simulink model "StopForInstabilityObserverForce"  (R2016b)
settings: configuration reference "WheelSimConfiguration2016" (kept outside this file)
libraries: simulink x1
settings Model: Creator=At  LastModifiedBy=ateay
settings ConfigSetRef: SourceLocation=Base Workspace

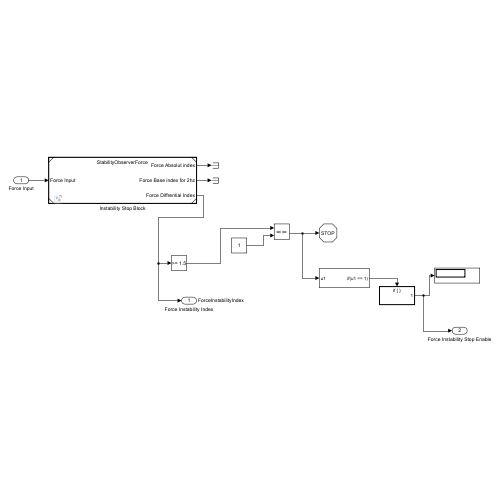
[thumbnail: Simulink's stored preview of the top-level diagram]
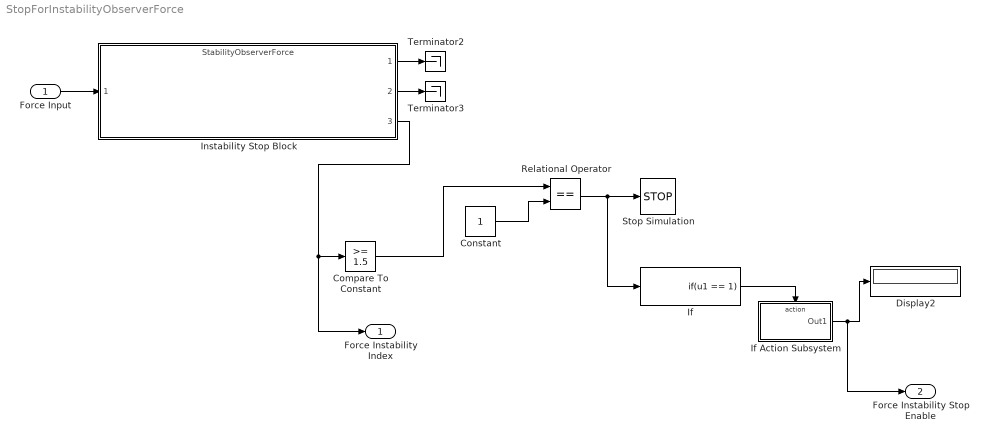
== system StopForInstabilityObserverForce ==
  Force Input : Inport
  Compare To Constant : simulink/Logic and Bit Operations/Compare To Constant  relop=>=  const=1.5  OutDataTypeStr=boolean
  Constant : Constant
  Display2 : Display
  If : If  IfExpression=u1 == 1  ShowElse=off
  If Action Subsystem : Subsystem  TreatAsAtomicUnit=on
  Instability Stop Block : ModelReference  ModelNameDialog=StabilityObserverForce.slx  SimulationMode=Normal  ModelReferenceVersion=1.20
  Relational Operator : RelationalOperator  Operator===  OutDataTypeStr=boolean  RndMeth=Simplest
  Stop Simulation : Stop
  Terminator2 : Terminator
  Terminator3 : Terminator
  Force Instability Index : Outport  SignalName=ForceInstabilityIndex
  Force Instability Stop Enable : Outport  Port=2
  wires:
  Instability Stop Block/3 -> Force Instability Index/1, Compare To Constant/1
  Compare To Constant/1 -> Relational Operator/1
  Constant/1 -> Relational Operator/2
  Relational Operator/1 -> If/1, Stop Simulation/1
  If/1 -> If Action Subsystem/Action
  If Action Subsystem/1(Out1) -> Force Instability Stop Enable/1, Display2/1
  Force Input/1 -> Instability Stop Block/1
  Instability Stop Block/1 -> Terminator2/1
  Instability Stop Block/2 -> Terminator3/1

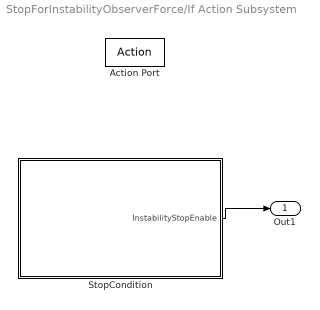
== system StopForInstabilityObserverForce/If Action Subsystem ==
  Action Port : ActionPort
  StopCondition : MATLAB Function  TreatAsAtomicUnit=on
  Out1 : Outport
  wires:
  StopCondition/1(InstabilityStopEnable) -> Out1/1

== matlab function StopForInstabilityObserverForce/If Action Subsystem/StopCondition ==
  data: InstabilityStopEnable output
function InstabilityStopEnable   = stopcondition(  )

%% This function calculates the wheel acceleration based on the simple dynamic model of propelling in a straight line


    
InstabilityStopEnable=1;
